simulink model "tri3"  (R2016b)
settings: Solver=VariableStepAuto  StartTime=0.0  StopTime=20  RelTol=1e-3
settings Model: Creator=Admin  LastModifiedBy=Admin

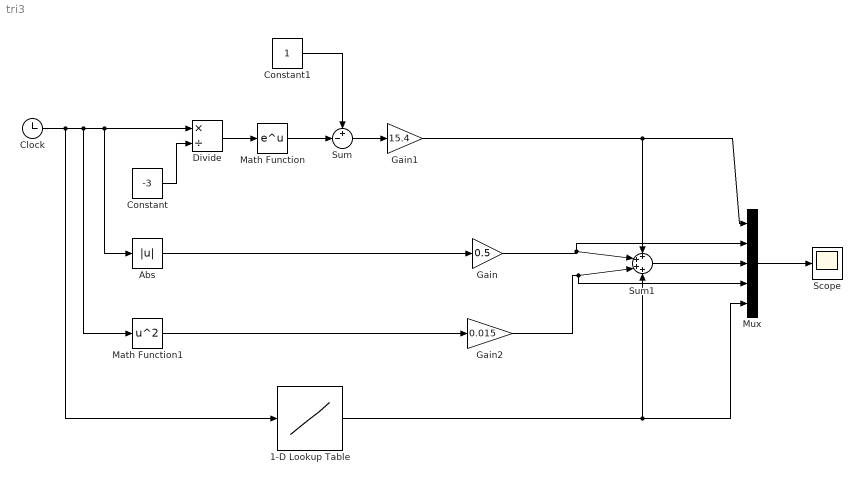
== system tri3 ==
  1-D Lookup Table : Lookup_n-D  NumberOfTableDimensions=1  BreakpointsForDimension1=[0,1.15,2.3,4.17,19.3,24.5]  Table=[0,1.3,3.1,6.2,11.15,25]  InternalRulePriority=Speed  RndMeth=Simplest  InputSameDT=on
  Abs : Abs
  Clock : Clock
  Constant : Constant  Value=-3
  Constant1 : Constant
  Divide : Product  Inputs=*/
  Gain : Gain  Gain=0.5
  Gain1 : Gain  Gain=15.4
  Gain2 : Gain  Gain=0.015
  Math Function : Math  SaturateOnIntegerOverflow=on
  Math Function1 : Math  Operator=square  SaturateOnIntegerOverflow=on
  Mux : Mux  Inputs=5
  Scope : Scope
  Sum : Sum  Inputs=+-|
  Sum1 : Sum  Inputs=++++
  wires:
  Clock/1 -> 1-D Lookup Table/1, Math Function1/1, Abs/1, Divide/1
  Constant/1 -> Divide/2
  Divide/1 -> Math Function/1
  Math Function/1 -> Sum/2
  Constant1/1 -> Sum/1
  Sum/1 -> Gain1/1
  Abs/1 -> Gain/1
  Math Function1/1 -> Gain2/1
  Mux/1 -> Scope/1
  1-D Lookup Table/1 -> Mux/5, Sum1/4
  Gain2/1 -> Mux/4, Sum1/3
  Gain/1 -> Mux/2, Sum1/2
  Gain1/1 -> Mux/1, Sum1/1
  Sum1/1 -> Mux/3
